simulink model "pitch_regulated_WT2"  (R2024b)
settings: Solver=FixedStepAuto  StartTime=0.0  StopTime=T_sim  FixedStep=dT  RelTol=1e-3
undefined symbols (not defined in the file): b, dT, inductance, Jeq, lambda_opt, magnets_flux, Noise_switch, noise_timeseries, omega_rotor_0, pole_pairs, R_rotor, rho_air, stat_resistance, switching_period, Trated, V_ci, V_co, V_rated, Vw_timeseries
libraries: slpidlib x3, simulink x1
settings Model: Creator=marti  LastModifiedBy=Andrea
settings DebuggingCC: AlgebraicLoopMsg=none
settings RTWCC: GPUComputeCapability=3.5

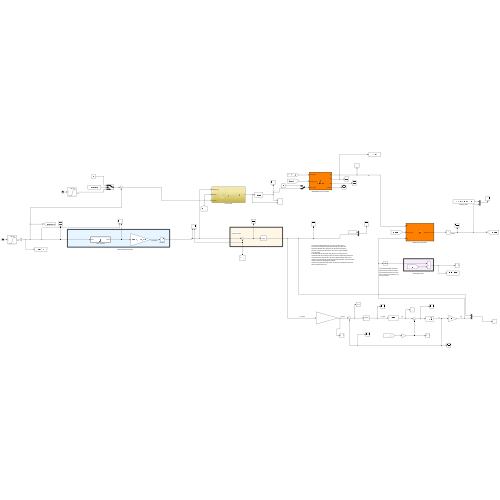
[thumbnail: Simulink's stored preview of the top-level diagram]
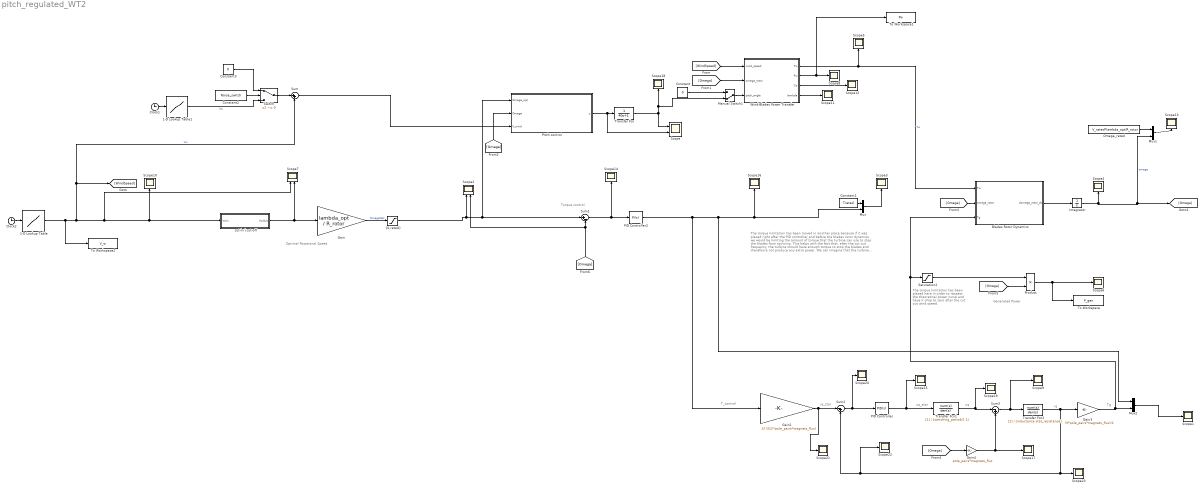
== system pitch_regulated_WT2 ==
  note: iq
  note: Tg
  note: uq
  note: uq_star
  note: iq_star
  note: T_control
  note: The torque limitation has been
      | placed here in order to respect
      | the theoretical power curve and
      | have it drop to zero after the cut
      | out wind speed.
  note: The torque limitation has been moved in another place
      | because if it was placed right after the PID controller and
      | before the blades rotor dynamics we would be limiting the
      | amount of torque that the turbine can use to stop the blades
      | from spinning.
      | This helps with the fact that, after the cut out frequency, the
      | turbine should have enough torque to stop the blades and therefoore
      | not produce any extra power. We can imagine that the turbine can
      | reach such high torques not just through the generator, but we assume
      | that the turbine is equipped with brakes.
      | However the generator and brakes torques are considered under the
      | same contritubution term
  note: Torque control
  note: Generated Power
  note: Optimal Rotational Speed
  1-D Lookup Table : Lookup_n-D  NumberOfTableDimensions=1  BreakpointsForDimension1=Vw_timeseries.Time  Table=Vw_timeseries.Data  InternalRulePriority=Speed  RndMeth=Simplest
  1-D Lookup Table1 : Lookup_n-D  NumberOfTableDimensions=1  BreakpointsForDimension1=noise_timeseries.Time  Table=noise_timeseries.Data  InternalRulePriority=Speed  RndMeth=Simplest
  Blades Rotor Dynamics : MATLAB Function  TreatAsAtomicUnit=on
  Clock1 : Clock
  Clock2 : Clock
  Constant : Constant  Value=0
  Constant1 : Constant  Value=Trated
  Constant2 : Constant  Value=Noise_switch
  Constant3 : Constant  Value=0
  Gain : Gain  Gain=lambda_opt / R_rotor
  Gain1 : Gain  Gain=1/((3/2)*pole_pairs*magnets_flux)
  Gain3 : Gain  Gain=(3*pole_pairs*magnets_flux)/2
  Gain4 : Gain  Gain=pole_pairs*magnets_flux
  Integrator : Integrator  InitialCondition=omega_rotor_0
  Manual Switch1 : ManualSwitch  CurrentSetting=0
  Mux : Mux  Inputs=2
  Mux1 : Mux  Inputs=2
  Mux2 : Mux  Inputs=2
  Omega_rated : Constant  Value=V_rated*lambda_opt/R_rotor
  PID Controller : slpidlib/PID Controller  Controller=PID  Form=Parallel  TimeDomain=Continuous-time  UseExternalTs=off  SampleTime=-1  IntegratorMethod=Forward Euler  FilterMethod=Forward Euler  ControllerParametersSource=internal  P=700  I=2  UseKiTs=off  D=0  UseExternalDerivativeSource=off  N=100  UseFilter=on  TunerSelectOption=Transfer Function Based (PID Tuner App)  InitialConditionSource=internal  InitialConditionForIntegrator=0  InitialConditionForFilter=0  DifferentiatorICPrevScaledInput=0  ExternalReset=none  TrackingMode=off  Kt=1  LimitOutput=off  SatLimitsSource=internal  UpperSaturationLimit=inf  LowerSaturationLimit=-inf  LinearizeAsGain=on  AntiWindupMode=none  Kb=1  LimitIntegrator=off  UpperIntegratorSaturationLimit=inf  LowerIntegratorSaturationLimit=-inf  POutMin=[]  POutMax=[]  IOutMin=[]  IOutMax=[]  DOutMin=[]  DOutMax=[]  NOutMin=[]  NOutMax=[]  SumOutMin=[]  SumOutMax=[]  SaturationOutMin=[]  SaturationOutMax=[]  PParamMin=[]  PParamMax=[]  IParamMin=[]  IParamMax=[]  DParamMin=[]  DParamMax=[]  NParamMin=[]  NParamMax=[]  KbParamMin=[]  KbParamMax=[]  KtParamMin=[]  KtParamMax=[]  KbOutMin=[]  KbOutMax=[]  KtOutMin=[]  KtOutMax=[]  IntegratorOutMin=[]  IntegratorOutMax=[]  FilterOutMin=[]  FilterOutMax=[]  SumI1OutMin=[]  SumI1OutMax=[]  SumI2OutMin=[]  SumI2OutMax=[]  SumI3OutMin=[]  SumI3OutMax=[]  SumI4OutMin=[]  SumI4OutMax=[]  SumDOutMin=[]  SumDOutMax=[]  DifferentiatorOutMin=[]  DifferentiatorOutMax=[]  FilterDiffOutCoefMin=[]  FilterDiffOutCoefMax=[]  ReciprocalOutMin=[]  ReciprocalOutMax=[]  SumDenOutMin=[]  SumDenOutMax=[]  SumNumOutMin=[]  SumNumOutMax=[]  DivideOutMin=[]  DivideOutMax=[]  UdiffTsProdOutMin=[]  UdiffTsProdOutMax=[]  NTsProdOutMin=[]  NTsProdOutMax=[]  UintegralTsProdOutMin=[]  UintegralTsProdOutMax=[]  UngainTsProdOutMin=[]  UngainTsProdOutMax=[]  ClampingZeroOutDataTypeStr=Inherit: Inherit via back propagation  ClampingZeroOutMin=[]  ClampingZeroOutMax=[]  FilterDenConstantOutDataTypeStr=Inherit: Inherit via back propagation  FilterDenConstantOutMin=[]  FilterDenConstantOutMax=[]  PCopyOutDataTypeStr=Inherit: Inherit via back propagation  PCopyOutMin=[]  PCopyOutMax=[]  NCopyOutDataTypeStr=Inherit: Inherit via back propagation  NCopyOutMin=[]  NCopyOutMax=[]  IntegratorContinuousStateAttributes=''  IntegratorStateMustResolveToSignalObject=off  IntegratorRTWStateStorageClass=Auto  FilterContinuousStateAttributes=''  FilterStateMustResolveToSignalObject=off  FilterRTWStateStorageClass=Auto  ParallelPVariant=InternalParameters  IdealPVariant=Disabled  IVariant=InternalParameters  DVariant=InternalParameters  IntegratorVariant=Continuous  SatVariant=Disabled  AWVariant=Passthrough  PCopyVariant=Disabled  TRVariant=Disabled  FdbkBlocksVariant=Forward  IdealPFdbkVariant=Disabled  SatFdbkVariant=Disabled  DerivativeFilterVariant=ContFilter  NVariant=InternalParameters  NCopyVariant=Disabled  FilterICVariant=InternalICsFilter  IntegratorICVariant=InternalICs  ExternalResetVariant=Disabled  TRSumVariant=Passthrough  SumFdbkVariant=Disabled  SumVariant=Sum_PID  TsampFilterVariant=InternalTs  TsampNgainVariant=Passthrough  TsampIntegralVariant=Disabled_SignalSpec  ExternalSaturationOutDataTypeStr=Inherit: Same as second input  DerivativeSourceVariant=ErrorSignal  PreIntVariant=InternalPreInt
  PID Controller2 : slpidlib/PID Controller  Controller=PI  Form=Parallel  TimeDomain=Continuous-time  UseExternalTs=off  SampleTime=-1  IntegratorMethod=Forward Euler  FilterMethod=Forward Euler  ControllerParametersSource=internal  P=-73149137.4852557  I=-4120963.14928724  UseKiTs=off  D=-26233555.3297944  UseExternalDerivativeSource=off  N=0.101497456028585  UseFilter=on  TunerSelectOption=Transfer Function Based (PID Tuner App)  InitialConditionSource=internal  InitialConditionForIntegrator=0  InitialConditionForFilter=0  DifferentiatorICPrevScaledInput=0  ExternalReset=none  TrackingMode=off  Kt=1  LimitOutput=off  SatLimitsSource=internal  UpperSaturationLimit=inf  LowerSaturationLimit=-inf  LinearizeAsGain=on  AntiWindupMode=none  Kb=1  LimitIntegrator=off  UpperIntegratorSaturationLimit=inf  LowerIntegratorSaturationLimit=-inf  POutMin=[]  POutMax=[]  IOutMin=[]  IOutMax=[]  DOutMin=[]  DOutMax=[]  NOutMin=[]  NOutMax=[]  SumOutMin=[]  SumOutMax=[]  SaturationOutMin=[]  SaturationOutMax=[]  PParamMin=[]  PParamMax=[]  IParamMin=[]  IParamMax=[]  DParamMin=[]  DParamMax=[]  NParamMin=[]  NParamMax=[]  KbParamMin=[]  KbParamMax=[]  KtParamMin=[]  KtParamMax=[]  KbOutMin=[]  KbOutMax=[]  KtOutMin=[]  KtOutMax=[]  IntegratorOutMin=[]  IntegratorOutMax=[]  FilterOutMin=[]  FilterOutMax=[]  SumI1OutMin=[]  SumI1OutMax=[]  SumI2OutMin=[]  SumI2OutMax=[]  SumI3OutMin=[]  SumI3OutMax=[]  SumI4OutMin=[]  SumI4OutMax=[]  SumDOutMin=[]  SumDOutMax=[]  DifferentiatorOutMin=[]  DifferentiatorOutMax=[]  FilterDiffOutCoefMin=[]  FilterDiffOutCoefMax=[]  ReciprocalOutMin=[]  ReciprocalOutMax=[]  SumDenOutMin=[]  SumDenOutMax=[]  SumNumOutMin=[]  SumNumOutMax=[]  DivideOutMin=[]  DivideOutMax=[]  UdiffTsProdOutMin=[]  UdiffTsProdOutMax=[]  NTsProdOutMin=[]  NTsProdOutMax=[]  UintegralTsProdOutMin=[]  UintegralTsProdOutMax=[]  UngainTsProdOutMin=[]  UngainTsProdOutMax=[]  ClampingZeroOutDataTypeStr=Inherit: Inherit via back propagation  ClampingZeroOutMin=[]  ClampingZeroOutMax=[]  FilterDenConstantOutDataTypeStr=Inherit: Inherit via back propagation  FilterDenConstantOutMin=[]  FilterDenConstantOutMax=[]  PCopyOutDataTypeStr=Inherit: Inherit via back propagation  PCopyOutMin=[]  PCopyOutMax=[]  NCopyOutDataTypeStr=Inherit: Inherit via back propagation  NCopyOutMin=[]  NCopyOutMax=[]  IntegratorContinuousStateAttributes=''  IntegratorStateMustResolveToSignalObject=off  IntegratorRTWStateStorageClass=Auto  FilterContinuousStateAttributes=''  FilterStateMustResolveToSignalObject=off  FilterRTWStateStorageClass=Auto  ParallelPVariant=InternalParameters  IdealPVariant=Disabled  IVariant=InternalParameters  DVariant=Disabled  IntegratorVariant=Continuous  SatVariant=Disabled  AWVariant=Passthrough  PCopyVariant=Disabled  TRVariant=Disabled  FdbkBlocksVariant=Forward  IdealPFdbkVariant=Disabled  SatFdbkVariant=Disabled  DerivativeFilterVariant=Disabled  NVariant=Disabled  NCopyVariant=Disabled_SignalSpec  FilterICVariant=Disabled  IntegratorICVariant=InternalICs  ExternalResetVariant=Disabled  TRSumVariant=Passthrough  SumFdbkVariant=Disabled  SumVariant=Sum_PI  TsampFilterVariant=InternalTs  TsampNgainVariant=Passthrough  TsampIntegralVariant=Disabled_SignalSpec  ExternalSaturationOutDataTypeStr=Inherit: Same as second input  DerivativeSourceVariant=Disabled  PreIntVariant=InternalPreInt
  Pitch control : Subsystem
  Product : Product
  Saturation2 : Saturate  UpperLimit=Trated  LowerLimit=-Inf
  Scope : Scope  NumInputPorts=2
  Scope{1,3..6,8..23} (21 alike) : Scope
  Scope2 : Scope  NumInputPorts=2
  Scope7 : Scope  NumInputPorts=2
  Sum : Sum  Inputs=|++
  Sum1 : Sum  Inputs=|+-
  Sum2 : Sum  Inputs=|-+
  Sum3 : Sum  Inputs=|-+
  Switch : Switch  Criteria=u2 ~= 0  SaturateOnIntegerOverflow=off  InputSameDT=off
  To Workspace : ToWorkspace  VariableName=P_gen  SampleTime=-1
      settings: Save2DSignal=2-D array (concatenate along first dimension)
  To Workspace1 : ToWorkspace  VariableName=Pw  SampleTime=-1
      settings: Save2DSignal=2-D array (concatenate along first dimension)
  To Workspace2 : ToWorkspace  VariableName=V_w  SampleTime=-1
      settings: Save2DSignal=2-D array (concatenate along first dimension)
  Transfer Fcn : TransferFcn  Denominator=[40 1]
  Transfer Fcn1 : TransferFcn  Denominator=[switching_period/2 1]
  Transfer Fcn2 : TransferFcn  Denominator=[inductance stat_resistance]
  Wind-Blades Power Transfer : MATLAB Function  TreatAsAtomicUnit=on
  cut-in | cut-off : MATLAB Function  TreatAsAtomicUnit=on
  "{0,rated}" : Saturate  UpperLimit=V_rated*lambda_opt/R_rotor  LowerLimit=0
  wires:
  Gain/1 -> "{0,rated}"/1  "OmegaOpt"
  [WindSpeed] -> Wind-Blades Power Transfer/1(wind_speed)
  Wind-Blades Power Transfer/1(Tw) -> Blades Rotor Dynamics/1(Tw), Scope5/1  "Tw"
  Blades Rotor Dynamics/1(domega_rotor_dt) -> Integrator/1
  Integrator/1 -> [Omega], Mux1/2, Scope4/1  "omega"
  [Omega] -> Wind-Blades Power Transfer/2(omega_rotor)
  [Omega] -> Blades Rotor Dynamics/2(omega_rotor)
  [Omega] -> Product/2
  Product/1 -> To Workspace/1, Scope6/1
  1-D Lookup Table/1 -> Scope7/1, cut-in | cut-off/1(VwIn), Scope10/1, Sum/2, [WindSpeed], To Workspace2/1  "Vw"
  "{0,rated}"/1 -> Scope2/1, Pitch control/1(Omega_opt), Sum1/1
  Wind-Blades Power Transfer/4(lambda) -> Scope11/1
  Wind-Blades Power Transfer/3(Cp) -> Scope12/1
  Manual Switch1/1 -> Wind-Blades Power Transfer/3(pitch_angle)
  Constant/1 -> Manual Switch1/1
  [Omega] -> Scope2/2, Sum1/2
  Wind-Blades Power Transfer/2(Pw) -> To Workspace1/1, Scope8/1
  Clock2/1 -> 1-D Lookup Table/1
  Constant1/1 -> Mux/1
  Mux/1 -> Scope3/1
  Omega_rated/1 -> Mux1/1
  Mux1/1 -> Scope13/1
  Sum1/1 -> PID Controller2/1, Scope14/1
  PID Controller2/1 -> Gain1/1, Mux2/1, Mux/2, Scope16/1
  [Omega] -> Pitch control/2(Omega)
  cut-in | cut-off/1(VwOut) -> Gain/1, Scope7/2
  Pitch control/1(y) -> Scope/2, Transfer Fcn/1
  Transfer Fcn/1 -> Scope/1, Scope18/1, Manual Switch1/2
  Constant2/1 -> Switch/2
  Clock1/1 -> 1-D Lookup Table1/1
  1-D Lookup Table1/1 -> Switch/3  "Vw"
  Constant3/1 -> Switch/1
  Switch/1 -> Sum/1
  Sum/1 -> Pitch control/3(V_wind)
  Saturation2/1 -> Product/1
  Gain1/1 -> Scope21/1, Sum2/1
  Sum2/1 -> Scope20/1, PID Controller/1
  PID Controller/1 -> Scope15/1, Transfer Fcn1/1
  Transfer Fcn1/1 -> Scope19/1, Sum3/1
  Sum3/1 -> Scope9/1, Transfer Fcn2/1
  [Omega] -> Gain4/1
  Gain4/1 -> Scope17/1, Sum3/2
  Mux2/1 -> Scope1/1
  Transfer Fcn2/1 -> Gain3/1, Scope22/1, Sum2/2, Scope23/1
  Gain3/1 -> Blades Rotor Dynamics/3(Tg), Saturation2/1, Mux2/2

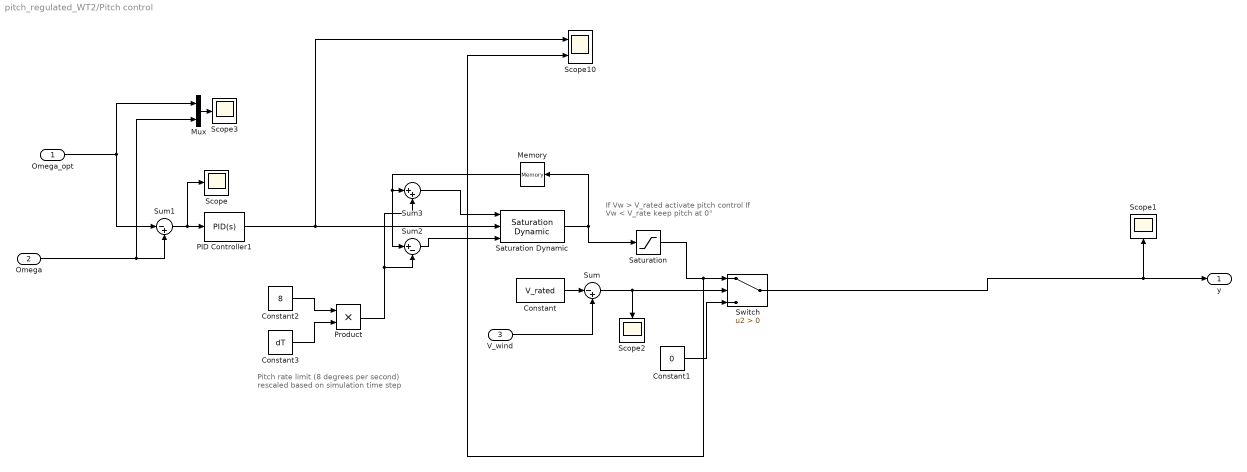
== system pitch_regulated_WT2/Pitch control ==
  note: Pitch rate limit (8 degrees per second)
      | rescaled based on simulation time step
  note: If Vw  >  V_rated activate pitch control
      | If Vw < V_rate keep pitch at 0°
  Omega_opt : Inport
  Omega : Inport  Port=2
  V_wind : Inport  Port=3
  Constant : Constant  Value=V_rated
  Constant1 : Constant  Value=0
  Constant2 : Constant  Value=8
  Constant3 : Constant  Value=dT
  Memory : Memory
  Mux : Mux  Inputs=2
  PID Controller1 : slpidlib/PID Controller  Controller=PID  Form=Parallel  TimeDomain=Continuous-time  UseExternalTs=off  SampleTime=-1  IntegratorMethod=Forward Euler  FilterMethod=Forward Euler  ControllerParametersSource=internal  P=1200  I=4  UseKiTs=off  D=10  UseExternalDerivativeSource=off  N=2  UseFilter=on  TunerSelectOption=Transfer Function Based (PID Tuner App)  InitialConditionSource=internal  InitialConditionForIntegrator=0  InitialConditionForFilter=0  DifferentiatorICPrevScaledInput=0  ExternalReset=none  TrackingMode=off  Kt=1  LimitOutput=off  SatLimitsSource=internal  UpperSaturationLimit=inf  LowerSaturationLimit=-inf  LinearizeAsGain=on  AntiWindupMode=none  Kb=1  LimitIntegrator=off  UpperIntegratorSaturationLimit=inf  LowerIntegratorSaturationLimit=-inf  POutMin=[]  POutMax=[]  IOutMin=[]  IOutMax=[]  DOutMin=[]  DOutMax=[]  NOutMin=[]  NOutMax=[]  SumOutMin=[]  SumOutMax=[]  SaturationOutMin=[]  SaturationOutMax=[]  PParamMin=[]  PParamMax=[]  IParamMin=[]  IParamMax=[]  DParamMin=[]  DParamMax=[]  NParamMin=[]  NParamMax=[]  KbParamMin=[]  KbParamMax=[]  KtParamMin=[]  KtParamMax=[]  KbOutMin=[]  KbOutMax=[]  KtOutMin=[]  KtOutMax=[]  IntegratorOutMin=[]  IntegratorOutMax=[]  FilterOutMin=[]  FilterOutMax=[]  SumI1OutMin=[]  SumI1OutMax=[]  SumI2OutMin=[]  SumI2OutMax=[]  SumI3OutMin=[]  SumI3OutMax=[]  SumI4OutMin=[]  SumI4OutMax=[]  SumDOutMin=[]  SumDOutMax=[]  DifferentiatorOutMin=[]  DifferentiatorOutMax=[]  FilterDiffOutCoefMin=[]  FilterDiffOutCoefMax=[]  ReciprocalOutMin=[]  ReciprocalOutMax=[]  SumDenOutMin=[]  SumDenOutMax=[]  SumNumOutMin=[]  SumNumOutMax=[]  DivideOutMin=[]  DivideOutMax=[]  UdiffTsProdOutMin=[]  UdiffTsProdOutMax=[]  NTsProdOutMin=[]  NTsProdOutMax=[]  UintegralTsProdOutMin=[]  UintegralTsProdOutMax=[]  UngainTsProdOutMin=[]  UngainTsProdOutMax=[]  ClampingZeroOutDataTypeStr=Inherit: Inherit via back propagation  ClampingZeroOutMin=[]  ClampingZeroOutMax=[]  FilterDenConstantOutDataTypeStr=Inherit: Inherit via back propagation  FilterDenConstantOutMin=[]  FilterDenConstantOutMax=[]  PCopyOutDataTypeStr=Inherit: Inherit via back propagation  PCopyOutMin=[]  PCopyOutMax=[]  NCopyOutDataTypeStr=Inherit: Inherit via back propagation  NCopyOutMin=[]  NCopyOutMax=[]  IntegratorContinuousStateAttributes=''  IntegratorStateMustResolveToSignalObject=off  IntegratorRTWStateStorageClass=Auto  FilterContinuousStateAttributes=''  FilterStateMustResolveToSignalObject=off  FilterRTWStateStorageClass=Auto  ParallelPVariant=InternalParameters  IdealPVariant=Disabled  IVariant=InternalParameters  DVariant=InternalParameters  IntegratorVariant=Continuous  SatVariant=Disabled  AWVariant=Passthrough  PCopyVariant=Disabled  TRVariant=Disabled  FdbkBlocksVariant=Forward  IdealPFdbkVariant=Disabled  SatFdbkVariant=Disabled  DerivativeFilterVariant=ContFilter  NVariant=InternalParameters  NCopyVariant=Disabled  FilterICVariant=InternalICsFilter  IntegratorICVariant=InternalICs  ExternalResetVariant=Disabled  TRSumVariant=Passthrough  SumFdbkVariant=Disabled  SumVariant=Sum_PID  TsampFilterVariant=InternalTs  TsampNgainVariant=Passthrough  TsampIntegralVariant=Disabled_SignalSpec  ExternalSaturationOutDataTypeStr=Inherit: Same as second input  DerivativeSourceVariant=ErrorSignal  PreIntVariant=InternalPreInt
  Product : Product
  Saturation : Saturate  UpperLimit=30  LowerLimit=0
  Saturation Dynamic : simulink/Discontinuities/Saturation Dynamic  OutMin=[]  OutMax=[]  OutDataTypeStr=Inherit: Same as second input  OutDataType=fixdt(1, 16)  OutScaling=2^-10  DoSatur=off
  Scope{,1..3} (4 alike) : Scope
  Scope10 : Scope  NumInputPorts=2
  Sum : Sum  Inputs=|-+
  Sum1 : Sum  Inputs=|-+
  Sum2 : Sum  Inputs=|+-
  Sum3 : Sum  Inputs=|++
  Switch : Switch  Criteria=u2 > Threshold  SaturateOnIntegerOverflow=off  InputSameDT=off
  y : Outport
  wires:
  PID Controller1/1 -> Scope10/1, Saturation Dynamic/2
  Omega/1 -> Mux/2, Sum1/2
  Omega_opt/1 -> Mux/1, Sum1/1
  Sum1/1 -> Scope/1, PID Controller1/1
  Saturation Dynamic/1 -> Memory/1, Saturation/1
  Constant1/1 -> Switch/3
  Sum/1 -> Switch/2, Scope2/1
  V_wind/1 -> Sum/2
  Constant/1 -> Sum/1
  Sum3/1 -> Saturation Dynamic/1
  Memory/1 -> Sum3/1, Sum2/1
  Sum2/1 -> Saturation Dynamic/3
  Constant2/1 -> Product/1
  Constant3/1 -> Product/2
  Product/1 -> Sum3/2, Sum2/2
  Saturation/1 -> Scope10/2, Switch/1
  Mux/1 -> Scope3/1
  Switch/1 -> Scope1/1, y/1

== matlab function pitch_regulated_WT2/cut-in | cut-off ==
  data: VwIn input; VwOut output; V_ci parameter; V_co parameter; V_rated parameter
function VwOut = fcn(VwIn,V_ci, V_co,V_rated)
if VwIn < V_ci
    VwOut = 0;
elseif VwIn >= V_ci && VwIn < V_co
    VwOut = VwIn;
else 
    VwOut = 0;
end

== matlab function pitch_regulated_WT2/Blades Rotor Dynamics ==
  data: Tw input; omega_rotor input; domega_rotor_dt output; Tg input; Jeq parameter; b parameter
  function domega_rotor_dt = fcn(Tw,omega_rotor,Tg,Jeq,b)

% Blades rotor shaft torques equilibrium:
% domega/dt * Jeq + b * omega = T_wind - T_generator

domega_rotor_dt = (Tw-Tg-b*omega_rotor)/Jeq;

== matlab function pitch_regulated_WT2/Wind-Blades Power Transfer ==
  data: wind_speed input; Tw output; omega_rotor input; pitch_angle input; R_rotor parameter; rho_air parameter; Pw output; Cp output; lambda output
function [Tw,Pw,Cp,lambda]   = WindTorque(wind_speed,omega_rotor,pitch_angle,R_rotor,rho_air)

fake_zero = 1e-6;
% Power Factor
lambda = omega_rotor*R_rotor/wind_speed;
Cp = PowerFactor(lambda,pitch_angle);
if Cp < fake_zero
    Cp = fake_zero;
end

% Wind power
Pw = 0.5 * rho_air * (pi * R_rotor^2) * Cp * wind_speed^3;

% Wind torque
Tw = Pw / omega_rotor;
